simulink model "m02b_linearization_model_comparison"  (R2021a)
settings: Solver=VariableStepAuto  StartTime=0.0  StopTime=20  RelTol=1e-3
values from neighbouring files (symbols this model uses):
  U0 = [0 0]    [linearization_data.mat]    (also in linearizedModel_Outputs.mat = [3.61873688012e-10 -3.90256021581e-22])
  Y0 = [0 0]    [linearization_data.mat]    (also in linearizedModel_Outputs.mat = [372.5 36.8372638482])
libraries: cstblocks x2, acolibjan22 x1
settings Model: Creator=e102261  LastModifiedBy=jason
settings SolverCC: AlgebraicLoopSolver=TrustRegion
settings DebuggingCC: ArithmeticOperatorsInVariantConditions=warning
settings SFSimCC: CustomCodeUndefinedFunction=UseInterfaceOnly

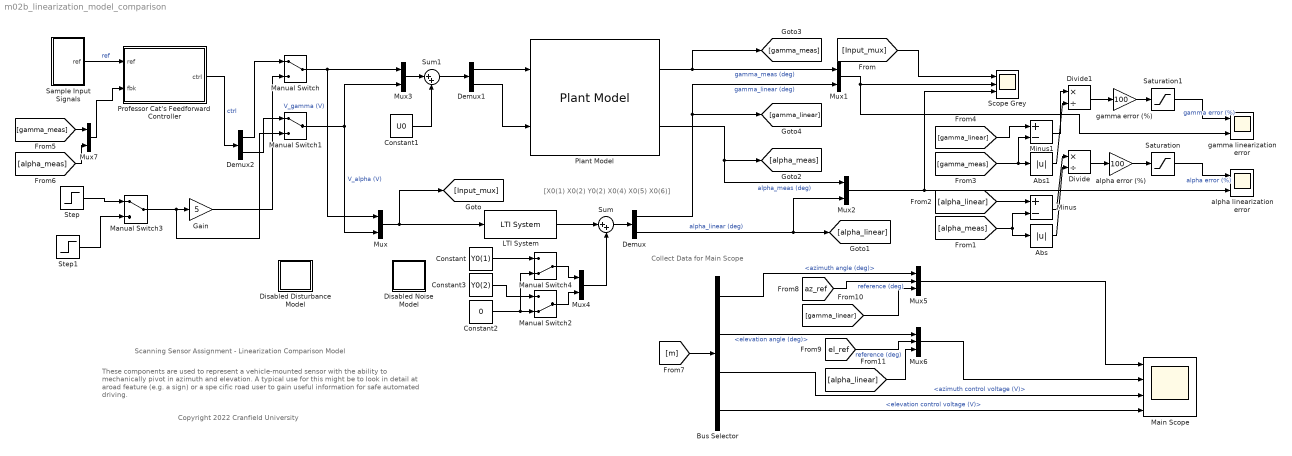
== system m02b_linearization_model_comparison ==
  note: [X0(1) X0(2) Y0(2) X0(4) X0(5) X0(6)]
  note: Collect Data for Main Scope
  note: These components are used to represent a vehicle-mounted sensor with the ability to mechanically pivot in azimuth and elevation.  A typical use for this might be to look in
      | detail at aroad feature (e.g. a sign) or a spe cific road user to gain useful information for
      | safe automated driving.
  note: Scanning Sensor Assignment - Linearization Comparison Model
  note: Copyright 2022 Cranfield University
  Abs : Abs
  Abs1 : Abs
  Bus Selector : BusSelector  OutputSignals=azimuth angle (deg),elevation angle (deg),azimuth control voltage (V),elevation control voltage (V)
  Constant : Constant  Value=Y0(1)
  Constant1 : Constant  Value=U0
  Constant2 : Constant  Value=0
  Constant3 : Constant  Value=Y0(2)
  Demux : Demux  Outputs=2
  Demux1 : Demux  Outputs=2
  Demux2 : Demux  Outputs=2
  Disabled Disturbance Model : Subsystem
      mask Display:
      | color('red');
      | fprintf('off')
  Disabled Noise Model : Subsystem
      mask Display:
      | color('red');
      | fprintf('off')
  Divide : Product  Inputs=*/
  Divide1 : Product  Inputs=*/
  Gain : Gain  Gain=5
  LTI System : cstblocks/LTI System  sys=P_ss_self  IC=[]
  Main Scope : Scope  NumInputPorts=4
  Manual Switch : ManualSwitch
  Manual Switch1 : ManualSwitch
  Manual Switch2 : ManualSwitch  CurrentSetting=0
  Manual Switch3 : ManualSwitch
  Manual Switch4 : ManualSwitch  CurrentSetting=0
  Minus : Sum  Inputs=+-
  Minus1 : Sum  Inputs=+-
  Mux{,1..4,7} (6 alike) : Mux  Inputs=2
  Mux5 : Mux  Inputs=3
  Mux6 : Mux  Inputs=3
  Plant Model : acolibjan22/Plant Model  X0=0
      settings: AttributesFormatString=Initial States = %<X0>
  Professor Cat's Feedforward Controller : Subsystem  LoadFcn=load feedforward_controller  InitFcn=load feedforward_controller
      settings: AttributesFormatString=Your controller replaces this!
      mask Display: image('graphic1.jpg')
  Sample Input Signals : Subsystem
  Saturation : Saturate  UpperLimit=200  LowerLimit=-200
  Saturation1 : Saturate  UpperLimit=200  LowerLimit=-200
  Scope Grey : Scope  NumInputPorts=3
  Step : Step  After=0.5  SampleTime=0
  Step1 : Step  After=-1.5  SampleTime=0
  Sum : Sum  Inputs=|++
  Sum1 : Sum  Inputs=|++
  alpha error (%) : Gain  Gain=100
  alpha linearization error : Scope  NumInputPorts=2
  gamma error (%) : Gain  Gain=100
  gamma linearization error : Scope  NumInputPorts=2
  wires:
  Manual Switch/1 -> Mux/1, Mux3/1  "V_gamma (V)"
  Plant Model/1 -> [gamma_meas], Mux1/1  "gamma_meas (deg)"
  Sum/1 -> Demux/1
  LTI System/1 -> Sum/1
  Constant/1 -> Manual Switch4/1
  Mux/1 -> LTI System/1, [Input_mux]
  [Input_mux] -> Scope Grey/1
  Demux/1 -> Mux1/2, [gamma_linear]  "gamma_linear (deg)"
  Demux/2 -> Mux2/2, [alpha_linear]  "alpha_linear (deg)"
  Mux1/1 -> Scope Grey/2, gamma linearization error/2
  Manual Switch1/1 -> Mux3/2, Mux/2  "V_alpha (V)"
  Gain/1 -> Manual Switch/2
  Mux3/1 -> Sum1/1
  Constant1/1 -> Sum1/2
  Sum1/1 -> Demux1/1
  Demux1/1 -> Plant Model/1
  Demux1/2 -> Plant Model/2
  Plant Model/2 -> [alpha_meas], Mux2/1  "alpha_meas (deg)"
  Constant2/1 -> Manual Switch4/2, Manual Switch2/2
  Mux4/1 -> Sum/2
  Constant3/1 -> Manual Switch2/1
  Manual Switch2/1 -> Mux4/2
  alpha error (%)/1 -> Saturation/1
  Mux2/1 -> Scope Grey/3, alpha linearization error/2
  Divide/1 -> alpha error (%)/1
  Minus/1 -> Divide/1
  [alpha_meas] -> Abs/1, Minus/2
  [alpha_linear] -> Minus/1
  Divide1/1 -> gamma error (%)/1
  [gamma_meas] -> Minus1/2, Abs1/1
  Minus1/1 -> Divide1/1
  [gamma_linear] -> Minus1/1
  gamma error (%)/1 -> Saturation1/1
  Saturation/1 -> alpha linearization error/1  "alpha error (%)"
  Saturation1/1 -> gamma linearization error/1  "gamma error (%)"
  Abs/1 -> Divide/2
  Abs1/1 -> Divide1/2
  Step1/1 -> Manual Switch3/2
  Manual Switch3/1 -> Manual Switch1/2, Gain/1
  Step/1 -> Manual Switch3/1
  Sample Input Signals/1(ref) -> Professor Cat's Feedforward Controller/1(ref)  "ref"
  Professor Cat's Feedforward Controller/1(ctrl) -> Demux2/1  "ctrl"
  Demux2/1 -> Manual Switch/1
  Demux2/2 -> Manual Switch1/1
  Bus Selector/4 -> Main Scope/4  "<elevation control voltage (V)>"
  Bus Selector/3 -> Main Scope/3  "<azimuth control voltage (V)>"
  Mux6/1 -> Main Scope/2
  [el_ref] -> Mux6/2  "reference (deg)"
  Bus Selector/2 -> Mux6/1  "<elevation angle (deg)>"
  Bus Selector/1 -> Mux5/1  "<azimuth angle (deg)>"
  Mux5/1 -> Main Scope/1
  [m] -> Bus Selector/1
  [gamma_meas] -> Mux7/1
  [alpha_meas] -> Mux7/2
  Mux7/1 -> Professor Cat's Feedforward Controller/2(fbk)
  [alpha_linear] -> Mux6/3
  [gamma_linear] -> Mux5/3
  [az_ref] -> Mux5/2  "reference (deg)"
  Manual Switch4/1 -> Mux4/1

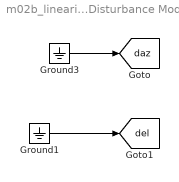
== system m02b_linearization_model_comparison/Disabled Disturbance Model ==
  Ground1 : Ground
  Ground3 : Ground
  tag scope: daz=global, del=global
  wires:
  Ground3/1 -> [daz]
  Ground1/1 -> [del]

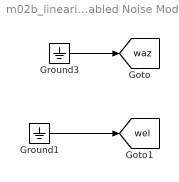
== system m02b_linearization_model_comparison/Disabled Noise Model ==
  Ground1 : Ground
  Ground3 : Ground
  tag scope: waz=global, wel=global
  wires:
  Ground1/1 -> [wel]
  Ground3/1 -> [waz]

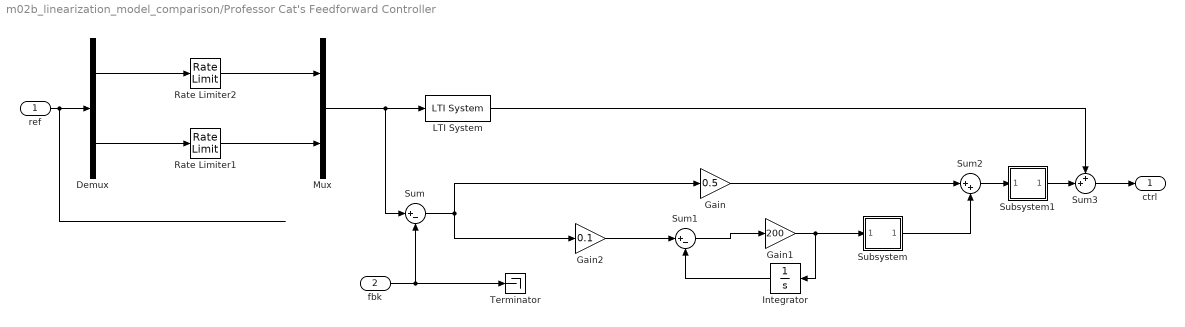
== system m02b_linearization_model_comparison/Professor Cat's Feedforward Controller ==
  ref : Inport
  fbk : Inport  Port=2
  Demux : Demux  Outputs=2
  Gain : Gain  Gain=0.5
  Gain1 : Gain  Gain=200
  Gain2 : Gain  Gain=0.1
  Integrator : Integrator
  LTI System : cstblocks/LTI System  sys=Qff  IC=[]
      settings: AttributesFormatString=|
      | This is a feedforward controller
      | which tries to invert out any
      | unwanted dynamics and replaces
      | them with the ones we do want.
  Mux : Mux  Inputs=2
  Rate Limiter1 : RateLimiter  RisingSlewLimit=55  FallingSlewLimit=-55
      settings: AttributesFormatString=|
      | RisingSlewLimit=%<RisingSlewLimit>
      | FallingSlewLimit=%<FallingSlewLimit>
      | 
      | Professor Cat found that these limits were
      | needed to make his feedforward controller
      | work at all.  Why?
      | 
      | Can you manage without them with feedback?
      | Can they still be helpful with feedback?
      | There isn't a unique answer here.
  Rate Limiter2 : RateLimiter  RisingSlewLimit=55  FallingSlewLimit=-55
      settings: AttributesFormatString=|
      | RisingSlewLimit=%<RisingSlewLimit>
      | FallingSlewLimit=%<FallingSlewLimit>
  Subsystem : Subsystem
  Subsystem1 : Subsystem
  Sum : Sum  Inputs=|+-
  Sum1 : Sum  Inputs=|+-
  Sum2 : Sum  Inputs=|++
  Sum3 : Sum  Inputs=++|
  Terminator : Terminator
      settings: AttributesFormatString=|
      | Professor Cat doesn't know about feedback
      | control so he has ignored the feedback signal.
      | Don't do this! :-)
  ctrl : Outport
  wires:
  fbk/1 -> Sum/2, Terminator/1
  LTI System/1 -> Sum3/1
  Demux/1 -> Rate Limiter2/1
  Mux/1 -> Sum/1, LTI System/1
  Demux/2 -> Rate Limiter1/1
  Rate Limiter2/1 -> Mux/1
  Rate Limiter1/1 -> Mux/2
  ref/1 -> Demux/1
  Sum/1 -> Gain2/1, Gain/1
  Gain/1 -> Sum2/1
  Gain1/1 -> Subsystem/1(In1), Integrator/1
  Integrator/1 -> Sum1/2
  Sum1/1 -> Gain1/1
  Sum2/1 -> Subsystem1/1(In1)
  Gain2/1 -> Sum1/1
  Subsystem/1(Out1) -> Sum2/2
  Subsystem1/1(ctrl) -> Sum3/2
  Sum3/1 -> ctrl/1

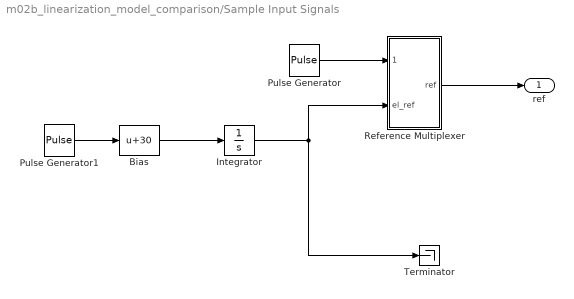
== system m02b_linearization_model_comparison/Sample Input Signals ==
  Bias : Bias  Bias=30
  Integrator : Integrator
  Pulse Generator : DiscretePulseGenerator  PulseType=Time based  Amplitude=35  Period=10  PulseWidth=50  PhaseDelay=1
  Pulse Generator1 : DiscretePulseGenerator  PulseType=Time based  Amplitude=-120/2  Period=4  PulseWidth=50  PhaseDelay=2
  Reference Multiplexer : Subsystem
      settings: AttributesFormatString=|
      | Contains global GOTO
      | blocks for logging
  Terminator : Terminator
      settings: AttributesFormatString=|
      | This is the elevation velocity
      | if you need it for state space
      | control setpoints.
  ref : Outport
  wires:
  Pulse Generator/1 -> Reference Multiplexer/1(az_ref)
  Reference Multiplexer/1(ref) -> ref/1
  Integrator/1 -> Terminator/1, Reference Multiplexer/2(el_ref)
  Pulse Generator1/1 -> Bias/1
  Bias/1 -> Integrator/1

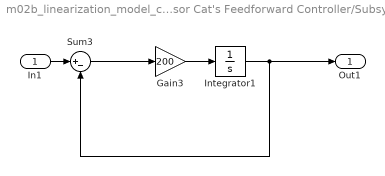
== system m02b_linearization_model_comparison/Professor Cat's Feedforward Controller/Subsystem ==
  In1 : Inport
  Gain3 : Gain  Gain=200
  Integrator1 : Integrator
  Sum3 : Sum  Inputs=|+-
  Out1 : Outport
  wires:
  Integrator1/1 -> Out1/1, Sum3/2
  Gain3/1 -> Integrator1/1
  Sum3/1 -> Gain3/1
  In1/1 -> Sum3/1

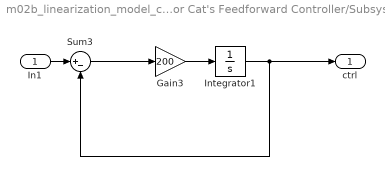
== system m02b_linearization_model_comparison/Professor Cat's Feedforward Controller/Subsystem1 ==
  In1 : Inport
  Gain3 : Gain  Gain=200
  Integrator1 : Integrator
  Sum3 : Sum  Inputs=|+-
  ctrl : Outport
  wires:
  In1/1 -> Sum3/1
  Sum3/1 -> Gain3/1
  Gain3/1 -> Integrator1/1
  Integrator1/1 -> Sum3/2, ctrl/1

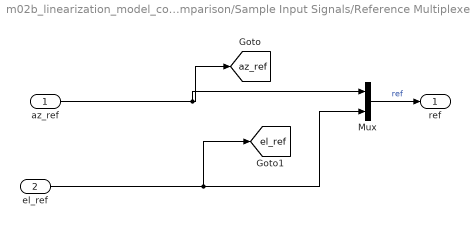
== system m02b_linearization_model_comparison/Sample Input Signals/Reference Multiplexer ==
  az_ref : Inport
  el_ref : Inport  Port=2
  Mux : Mux  Inputs=2
  ref : Outport
  tag scope: az_ref=global, el_ref=global
  wires:
  Mux/1 -> ref/1  "ref"
  az_ref/1 -> Mux/1, [az_ref]
  el_ref/1 -> Mux/2, [el_ref]
